simulink model "mod_bpsk"  (Simulink 7.2)
settings: Solver=FixedStepDiscrete  StartTime=0.0  StopTime=inf  RelTol=1e-3
InitFcn:
  | mod_bpsk_m
values from neighbouring files (symbols this model uses):
  frame = 128    [mod_bpsk_m.m]
  N_samples = K * of    (= 32)    [mod_bpsk_m.m]
  Tb = N_samples*Tc    (= 0.000725623582766)    [mod_bpsk_m.m]
  Tc = 1/fc    (= 2.26757369615e-05)    [mod_bpsk_m.m]
undefined symbols (not defined in the file or in its folder): Fs, get
libraries: dspsnks4 x4, commdigbbndpm3 x1, commrandsrc2 x1, commsink2 x1, commfilt2 x1, dspsrcs4 x1
settings Model: Creator=Francesco Pizzo  LastModifiedBy=Francesco

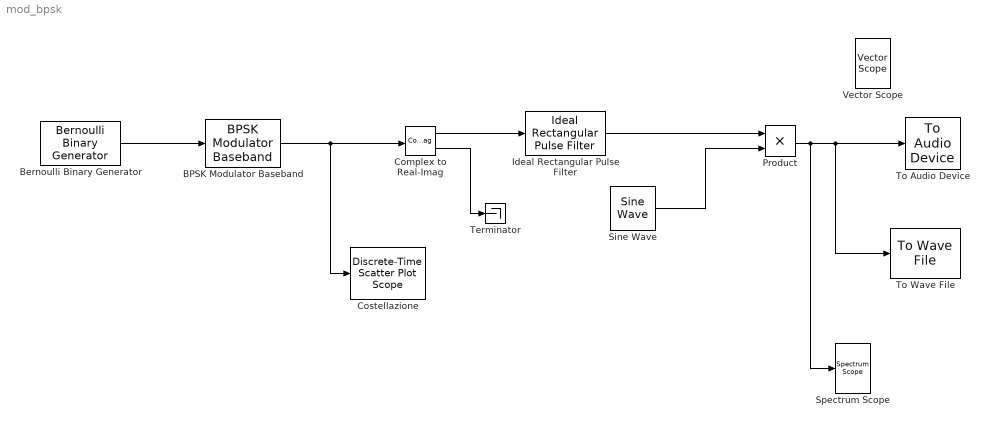
== system mod_bpsk ==
  BPSK Modulator Baseband : commdigbbndpm3/BPSK Modulator Baseband  DialogController=commDDGCreate  DialogControllerArgs=DataTag0  SystemSampleTime=-1  Ph=0  outDtype=double  outWordLen=16  outUDDataType=sfix(16)  outFracLenMode=Best precision  outFracLen=15
  Bernoulli Binary Generator : commrandsrc2/Bernoulli Binary Generator  DialogController=commDDGCreate  DialogControllerArgs=DataTag1  SystemSampleTime=-1  P=0.5  seed=randseed  Ts=Tb  frameBased=on  sampPerFrame=frame  orient=off  outDataType=double
  Complex to Real-Imag : ComplexToRealImag
  Costellazione : commsink2/Discrete-Time Scatter Plot Scope  Tag=ScatterPlot  SystemSampleTime=-1  sampPerSymb=1  offsetEye=0  numTraces=40  numNewFrames=10  LineMarkers=x  LineColors=k  fading=on  render=on  AxisGrid=on  xMin=-3.3  xMax=3.315  yMin=-3.3  yMax=3.315  inphaseLabel=In-phase Amplitude  quadratureLabel=Quadrature Amplitude  openScopeAtSimStart=on  FrameNumber=off  FigPos=get(0,'defaultfigureposition');  figTitle=Scatter Plot  numLinesMax=8  block_type_=scatter
  Ideal Rectangular Pulse Filter : commfilt2/Ideal Rectangular Pulse Filter  DialogController=commDDGCreate  DialogControllerArgs=DataTag2  SystemSampleTime=-1  pulseLen=N_samples  pulseDelay=0  sampMode=Frame-based  normCheck=off  normMode=Sum of samples  filterGain=1  roundingMode=Floor  overflowMode=off
  Product : Product  OutDataType=sfix(16)  OutScaling=2^0  RndMeth=Zero
  Sine Wave : dspsrcs4/Sine Wave  Amplitude=1  Frequency=1e4  Phase=pi/2  SampleMode=Discrete  OutComplex=Real  CompMethod=Trigonometric fcn  TableSize=Speed  SampleTime=Tc  SamplesPerFrame=N_samples*frame  dataType=double  wordLen=16  udDataType=sfix(16)  fracBitsMode=Best precision  numFracBits=15  ResetState=Restart at time zero
  Spectrum Scope : dspsnks4/Spectrum Scope  DialogController=dspdialog.SpectrumScope  DialogControllerArgs=DataTag3  SystemSampleTime=-1  ScopeProperties=on  Domain=Frequency  HorizSpan=1  UseBuffer=off  BufferSize=128  Overlap=64  inpFftLenInherit=off  FFTlength=128  numAvg=2  DisplayProperties=off  AxisGrid=on  Memory=off  FrameNumber=on  AxisLegend=off  AxisZoom=off  OpenScopeAtSimStart=on  OpenScopeImmediately=off  FigPos=get(0,'defaultfigureposition')  AxisProperties=off  XUnits=Hertz  XRange=[-Fs/2...Fs/2]  XDisplay=0  InheritXIncr=off  XIncr=Tc  XLabel=Samples  XLimit=Auto  YUnits=dB  XMax=1  XMin=0  YLabel=Magnitude-squared, dB  LineProperties=off  wintypeSpecScope=Hann  RsSpecScope=50  betaSpecScope=5  winsampSpecScope=Periodic
      settings: YMin=-49.7646998299811  YMax=14.0893682951059
  Terminator : Terminator
  To Audio Device : dspsnks4/To Audio Device  DialogController=dspDDGCreate  DialogControllerArgs=DataTag4  deviceName=Default  inheritSampleRate=on  sampleRate=44100  deviceDatatype=Determine from input data type  autoBufferSize=on  bufferSize=4096  queueDuration=1.0
  To Wave File : dspsnks4/To Wave File  filename=bpsk  sampleWidth=16  MinNumSamples=256
  Vector Scope : dspsnks4/Vector Scope  DialogController=dspdialog.VectorScope  DialogControllerArgs=DataTag5  ScopeProperties=on  Domain=Time  HorizSpan=1  DisplayProperties=off  AxisGrid=on  Memory=off  FrameNumber=on  AxisLegend=off  AxisZoom=off  OpenScopeAtSimStart=on  OpenScopeImmediately=off  FigPos=get(0,'defaultfigureposition')  AxisProperties=off  XUnits=Hertz  XRange=[0...Fs/2]  InheritXIncr=on  XIncr=1  XLabel=Time  XLimit=Auto  XMin=0  XMax=1  XStart=0  YUnits=dB  YLabel=Amplitude  LineProperties=off
      settings: YMin=-1.05  YMax=1.05
  wires:
  Bernoulli Binary Generator/1 -> BPSK Modulator Baseband/1
  Complex to Real-Imag/1 -> Ideal Rectangular Pulse Filter/1
  BPSK Modulator Baseband/1 -> Complex to Real-Imag/1, Costellazione/1
  Complex to Real-Imag/2 -> Terminator/1
  Ideal Rectangular Pulse Filter/1 -> Product/1
  Sine Wave/1 -> Product/2
  Product/1 -> To Audio Device/1, To Wave File/1, Spectrum Scope/1
